simulink model "Navigation_Real"  (R2024a)
settings: Solver=VariableStepAuto  StartTime=0.0  StopTime=10.0  RelTol=1e-3
undefined symbols (not defined in the file or in its folder): Desired_Year_IGRF, Velocity_Ship_Mean
libraries: simulink_extras x4, sensorgpslib x1, sensorinslib x1
settings Model: Creator=gerar  LastModifiedBy=gerar

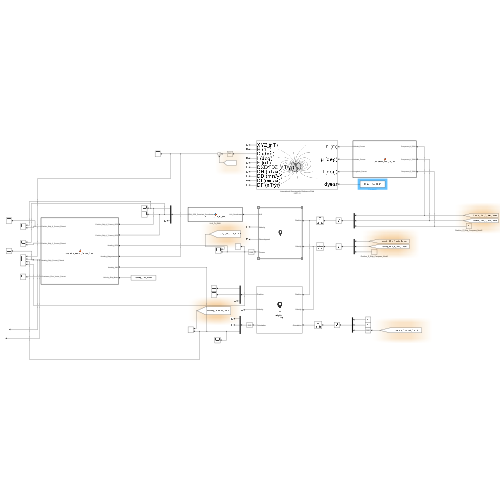
[thumbnail: Simulink's stored preview of the top-level diagram]
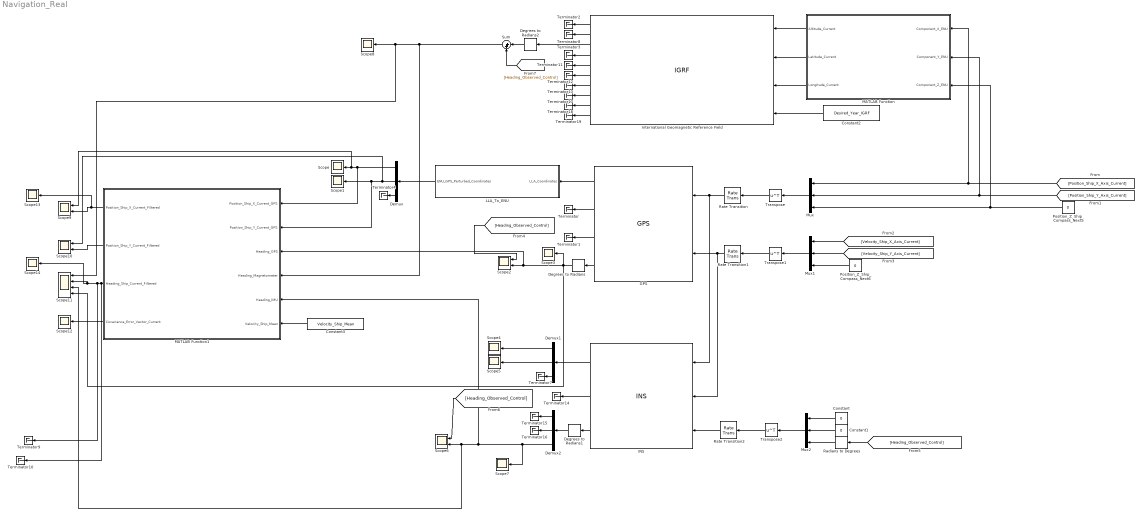
== system Navigation_Real ==
  Constant : Constant  Value=0
  Constant1 : Constant  Value=0
  Constant2 : Constant  Value=Desired_Year_IGRF
  Constant3 : Constant  Value=Velocity_Ship_Mean
  Degrees to Radians : simulink_extras/Transformations/Degrees to Radians
  Degrees to Radians1 : simulink_extras/Transformations/Degrees to Radians
  Degrees to Radians2 : simulink_extras/Transformations/Degrees to Radians
  Demux : Demux  Outputs=3
  Demux1 : Demux  Outputs=3
  Demux2 : Demux  Outputs=3
  GPS : sensorgpslib/GPS  DispRefFrame=ENU  PositionInputFormat=Local  ReferenceLocation=[43.059023, 3.002915 ,0]  HorizontalPositionAccuracy=1.6  VerticalPositionAccuracy=3  VelocityAccuracy=0.1  DecayFactor=0.999  SeedDouble=67  SimulateUsing=Interpreted execution
  INS : sensorinslib/INS  MountingLocation=[0 0 0]  RollAccuracy=0.2  PitchAccuracy=0.2  YawAccuracy=1  PositionAccuracy=1  VelocityAccuracy=0.05  UseAccelAndAngVel=off  AccelerationAccuracy=0  AngularVelocityAccuracy=0  TimeInput=off  PositionErrorFactor=[0 0 0]  SeedDouble=67  SimulateUsing=Code generation
  International Geomagnetic Reference Field : IGRF  month=January  day=1  year=2020
      settings: AttributesFormatString=%<generation>
  LLA_To_ENU : MATLAB Function  TreatAsAtomicUnit=on
  MATLAB Function : MATLAB Function  TreatAsAtomicUnit=on
  MATLAB Function1 : MATLAB Function  TreatAsAtomicUnit=on
  Mux : Mux  Inputs=3
  Mux1 : Mux  Inputs=3
  Mux2 : Mux  Inputs=3
  Position_Z_Ship_Compass_Next5 : Constant  Value=0
  Position_Z_Ship_Compass_Next6 : Constant  Value=0
  Radians to Degrees : simulink_extras/Transformations/Radians to Degrees
  Rate Transition : RateTransition  OutPortSampleTime=0.01
  Rate Transition1 : RateTransition  OutPortSampleTime=0.01
  Rate Transition2 : RateTransition  OutPortSampleTime=0.01
  Scope{,1,3..5,7..8,12..14} (10 alike) : Scope
  Scope{2,6,9..10} (4 alike) : Scope  NumInputPorts=2
  Scope11 : Scope  NumInputPorts=4
  Sum : Sum  Inputs=|++
  Terminator{,1..4,7..19} (18 alike) : Terminator
  Transpose : Math  Operator=transpose
  Transpose1 : Math  Operator=transpose
  Transpose2 : Math  Operator=transpose
  wires:
  MATLAB Function/1(Altitude_Current) -> International Geomagnetic Reference Field/1
  Demux/3 -> Terminator4/1
  International Geomagnetic Reference Field/6 -> Terminator12/1
  International Geomagnetic Reference Field/2 -> Terminator8/1
  Constant1/1 -> Mux2/2
  Transpose2/1 -> Rate Transition2/1
  Mux2/1 -> Transpose2/1
  Degrees to Radians1/1 -> Demux2/1
  [Heading_Observed_Control] -> Scope6/1
  MATLAB Function/3(Longitude_Current) -> International Geomagnetic Reference Field/3
  GPS/4 -> Degrees to Radians/1
  INS/3 -> Degrees to Radians1/1
  GPS/1 -> LLA_To_ENU/1(LLA_Coordinates)
  Demux1/1 -> Scope4/1
  Demux1/2 -> Scope5/1
  [Velocity_Ship_X_Axis_Current] -> Mux1/1
  Demux1/3 -> Terminator7/1
  [Position_Ship_Y_Axis_Current] -> MATLAB Function/2(Component_Y_ENU), Mux/2
  Degrees to Radians/1 -> MATLAB Function1/3(Heading_GPS), Scope2/2, Scope11/4, Scope3/1
  Demux/2 -> Scope10/1, MATLAB Function1/2(Position_Ship_Y_Current_GPS), Scope1/1
  [Heading_Observed_Control] -> Scope2/1
  Position_Z_Ship_Compass_Next6/1 -> Mux1/3
  Position_Z_Ship_Compass_Next5/1 -> MATLAB Function/3(Component_Z_ENU), Mux/3
  [Velocity_Ship_Y_Axis_Current] -> Mux1/2
  [Position_Ship_X_Axis_Current] -> MATLAB Function/1(Component_X_ENU), Mux/1
  Rate Transition/1 -> INS/1, GPS/1
  Transpose1/1 -> Rate Transition1/1
  International Geomagnetic Reference Field/3 -> Degrees to Radians2/1
  International Geomagnetic Reference Field/4 -> Terminator3/1
  International Geomagnetic Reference Field/9 -> Terminator18/1
  Rate Transition1/1 -> INS/2, GPS/2
  Constant/1 -> Mux2/1
  Mux/1 -> Transpose/1
  INS/2 -> Terminator14/1
  Sum/1 -> MATLAB Function1/4(Heading_Magnetometer), Scope11/1, Scope8/1
  [Heading_Observed_Control] -> Radians to Degrees/1
  International Geomagnetic Reference Field/7 -> Terminator13/1
  International Geomagnetic Reference Field/10 -> Terminator19/1
  International Geomagnetic Reference Field/8 -> Terminator17/1
  Demux2/2 -> Terminator16/1
  International Geomagnetic Reference Field/5 -> Terminator11/1
  International Geomagnetic Reference Field/1 -> Terminator2/1
  MATLAB Function/2(Latitude_Current) -> International Geomagnetic Reference Field/2
  Demux2/3 -> Scope7/1, Scope11/3, Scope6/2, MATLAB Function1/5(Heading_IMU)
  Transpose/1 -> Rate Transition/1
  INS/1 -> Demux1/1
  Demux/1 -> MATLAB Function1/1(Position_Ship_X_Current_GPS), Scope9/1, Scope/1
  Degrees to Radians2/1 -> Sum/1
  GPS/3 -> Terminator1/1
  Constant2/1 -> International Geomagnetic Reference Field/4
  Radians to Degrees/1 -> Mux2/3
  LLA_To_ENU/1(ENU_GPS_Perturbed_Coordinates) -> Demux/1
  MATLAB Function1/4(Covariance_Error_Vector_Current) -> Scope12/1
  Rate Transition2/1 -> INS/3
  Demux2/1 -> Terminator15/1
  GPS/2 -> Terminator/1
  MATLAB Function1/2(Position_Ship_Y_Current_Filtered) -> Scope10/2
  Mux1/1 -> Transpose1/1
  Constant3/1 -> MATLAB Function1/6(Velocity_Ship_Mean)
  MATLAB Function1/1(Position_Ship_X_Current_Filtered) -> Scope13/1, Scope9/2
  [Heading_Observed_Control] -> Sum/2
  MATLAB Function1/3(Heading_Ship_Current_Filtered) -> Terminator10/1, Terminator9/1, Scope14/1, Scope11/2

== matlab function Navigation_Real/LLA_To_ENU ==
  data: LLA_Coordinates input; ENU_GPS_Perturbed_Coordinates output
function ENU_GPS_Perturbed_Coordinates = Conversion_LLA_To_ENU(LLA_Coordinates)

% Reference point:
Reference_Point_Port_Mahon = [43.059023,3.002915,0];
Semi_Major_Axis = 6378137.0;
Flattening = 1/298.25;

% This function serves as a mean to convert LLA coordinates to ENU
% coordinates:
ENU_GPS_Perturbed_Coordinates = LLA_To_ENU(LLA_Coordinates(1),LLA_Coordinates(2),LLA_Coordinates(3),...
                                           Reference_Point_Port_Mahon(1),Reference_Point_Port_Mahon(2),...
                                           Reference_Point_Port_Mahon(3),Semi_Major_Axis,Flattening);


end

== matlab function Navigation_Real/MATLAB Function ==
  data: Altitude_Current output; Latitude_Current output; Longitude_Current output; Component_X_ENU input; Component_Y_ENU input; Component_Z_ENU input
function [Altitude_Current,Latitude_Current,Longitude_Current] = Conversion_ENU_To_LAA(Component_X_ENU,...
                                                                                       Component_Y_ENU,...
                                                                                       Component_Z_ENU)

% This function serves as a mean to convert ENU coordinates into LLA
% coordinates. Need to write an embedded function to be injected in the
% Mission Software.
% Reference point for the current mission;
Reference_Point_Port_Mahon = [43.059023,3.002915,0];
Position_Vector_ENU_Current = [Component_X_ENU,Component_Y_ENU,Component_Z_ENU];

% Conversion using Matlab function:
Position_Vector_LLA_Current = enu2lla(Position_Vector_ENU_Current,Reference_Point_Port_Mahon,'ellipsoid');

% Feed the outputs:
Latitude_Current = Position_Vector_LLA_Current(1);
Altitude_Current = Position_Vector_LLA_Current(3);
Longitude_Current = Position_Vector_LLA_Current(2);

end

== matlab function Navigation_Real/MATLAB Function1 ==
  data: Position_Ship_X_Current_GPS input; Position_Ship_Y_Current_GPS input; Heading_GPS input; Heading_Magnetometer input; Heading_IMU input; Position_Ship_X_Current_Filtered output; Position_Ship_Y_Current_Filtered output; Heading_Ship_Current_Filtered output; Covariance_Error_Vector_Current output; Velocity_Ship_Mean input
function [Position_Ship_X_Current_Filtered,...
          Position_Ship_Y_Current_Filtered,...
          Heading_Ship_Current_Filtered,...
          Covariance_Error_Vector_Current]  = Navigation_Kalman_Sensor_Fusion(Position_Ship_X_Current_GPS,...
                                                                              Position_Ship_Y_Current_GPS,...
                                                                              Heading_GPS,...
                                                                              Heading_Magnetometer,...
                                                                              Heading_IMU,...
                                                                              Velocity_Ship_Mean)

% This function serves as a filterting and data fusion to provide the ship
% with the right heading data.

% Openwork modifications:
% - Include the position given by the IMU if needed.
% - Complexification of the state model.

% ----------------------------------------------------------------
% 1) Definition of the process model:
% ----------------------------------------------------------------
% We define the following process model state vector:
% States_Initial_Model = [Position_X_Current;...
%                   Position_Y_Current;...
%                   Psi_Heading_Current;...
%                   Velocity_Current];

% Initialization of the current models:
Position_Ship_X_Current_Model = Position_Ship_X_Current_GPS;
Position_Ship_Y_Current_Model = Position_Ship_Y_Current_GPS;
Heading_Current_Model = Heading_GPS;
Velocity_Ship_Model = Velocity_Ship_Mean;

States_Initial_Model = [Position_Ship_X_Current_Model;...
                        Position_Ship_Y_Current_Model;...
                        Heading_Current_Model;...
                        Velocity_Ship_Model];

% We then define the process noise covariance matrix refered as the 'Q'
% matrix in estimation. This has a link with how one is confident about the
% used model:
Variance_Position_X = 0.5;
Variance_Position_Y = 0.5;
Variance_Heading = (2*pi/180);
Variance_Velocity = 10e-4;
Process_Model_Covariance_Matrix = [Variance_Position_X^2 0 0 0;
                                   0 Variance_Position_Y^2 0 0;
                                   0 0 Variance_Heading^2 0;
                                   0 0 0 Variance_Velocity^2];

% We define the covariance matrix of the states at the initial step refered as the 'P0|0':
% We just take Covariance_Matrix_States_Initial_Model =
% Process_Model_Covariance_Matrix:
Covariance_States_Initial_Model = Process_Model_Covariance_Matrix;

% Define the control input matrix refered as the 'B' matrix in the usual
% description of linear state-space system reprezentation:
Control_Inputs_Initial = 0; % Process model considered as without input influence.

% Chose the step time, it shall be aligned with HW specification:
Time_Step_HW = 1;

% NOTA:
% When calling the EKF function such that Estimates = EKF(), to get the
% proper evaluated functions used inside (Jacobians for example), then use
% the notation Estimates = EKF(Jacobian(Variable1,Variable2)).
% If it's not working, then delete the function as an input of the EKF,
% call it directly inside the EKF function. But pay attention to get the
% good inputs inside the EKF function.
% /!\ Same thing for the Function_Process_Model inside the EKF /!\.

% ----------------------------------------------------------------
% 2) Measurement & Innovation model:
% ----------------------------------------------------------------
% We define the following measurement model state vector:
% Measurement_Vector = [Position_X_Current;...
%                       Position_Y_Current;...
%                       Psi_Heading_GNSS_Current;...
%                       Psi_Heading_Mag_Current;...
%                       Psi_Heading_IMU_Current
%                       Velocity_Current];

% Definition of the measurement noise covariance matrix refered as 'R' matrix:
% Retake the Variance_Position_X, Variance_Position_Y, Variance_Velocity
% and Variance_Heading for Variance_Heading_GNSS used in the process model section:
% To be aligned with the specification from the sensors and the models used
% for the Navigation:
Variance_Position_X_GPS = 1.5;
Variance_Position_Y_GPS = 1;
Variance_Heading_GNSS = 6*(pi/180);
Variance_Heading_Magnetic = 10*(pi/180);
Variance_Heading_IMU = 15*(pi/180);
Measurement_Covariance_Matrix = [Variance_Position_X_GPS 0 0 0 0 0;
                                 0 Variance_Position_Y_GPS 0 0 0 0;
                                 0 0 Variance_Heading_GNSS 0 0 0;
                                 0 0 0 Variance_Heading_Magnetic 0 0;
                                 0 0 0 0 Variance_Heading_IMU 0;
                                 0 0 0 0 0 Variance_Velocity];

% Define the measurement model matrix: (ofter refered as 'H' or 'Gx'
% matrices):
Measurement_Model_Matrix = [1 0 0 0;
                            0 1 0 0;
                            0 0 1 0;
                            0 0 1 0;
                            0 0 1 0;
                            0 0 0 1];

% ----------------------------------------------------------------
% Extended Kalman Filter loop calculations:
% ----------------------------------------------------------------
% Store the results:
% States_Estimated_EKF = [];
% Covariance_Estimated_EKF = [];

% Initialization:
States_Previous = States_Initial_Model; % The 'X' state vector.
Covariance_State_Previous = Covariance_States_Initial_Model; % The 'P0|0' equal to 'Q' in this case.
Control_Inputs_Previous = Control_Inputs_Initial; % The usual 'B' matrix but unused here.
Process_Model_Covariance_Matrix_Previous = Process_Model_Covariance_Matrix; % The 'Q' process model matrix.
Measurement_Covariance_Matrix_Previous = Measurement_Covariance_Matrix; % The 'R' measurement matrix.
Measurment_Current = [Position_Ship_X_Current_GPS,Position_Ship_Y_Current_GPS,Heading_GPS,Heading_Magnetometer,...
                      Heading_IMU,Velocity_Ship_Mean];

% EKF loop calculation:
[State_Aposteriori_Current,Covariance_Aposteriori_Current] = EKF_Heading(States_Previous,Covariance_State_Previous,Control_Inputs_Previous,...
                                                                         Jacobian_State_Process_Model(States_Previous(4),States_Previous(3),Time_Step_HW),...
                                                                         Process_Model_Covariance_Matrix_Previous,Measurement_Model_Matrix,...
                                                                         Measurement_Covariance_Matrix_Previous,...
                                                                         Function_Process_Model(States_Previous(1),States_Previous(2),States_Previous(3),States_Previous(4),Time_Step_HW),...
                                                                         Measurment_Current');


% Inputs update:
% States_Initial_Model = State_Aposteriori_Current;
% Covariance_States_Initial_Model = Covariance_Aposteriori_Current;

% % Store the results:
% States_Estimated_EKF = [States_Estimated_EKF,State_Aposteriori_Current];
% Covariance_Estimated_EKF = [Covariance_Estimated_EKF,Covariance_Aposteriori_Current];

% Store the interesting components of the covariance matrix (diagonal
% terms):
Covariance_Position_X = Covariance_Aposteriori_Current(1,1);
Covariance_Position_Y = Covariance_Aposteriori_Current(2,2);
Covariance_Psi_Heading = Covariance_Aposteriori_Current(3,3);
Covariance_Velocity = Covariance_Aposteriori_Current(4,4);
Covariance_Error_Vector_Current = [Covariance_Position_X;...
                                   Covariance_Position_Y;...
                                   Covariance_Psi_Heading;...
                                   Covariance_Velocity];

% Filtered and fused data:
Position_Ship_X_Current_Filtered = State_Aposteriori_Current(1);
Position_Ship_Y_Current_Filtered = State_Aposteriori_Current(2);
Heading_Ship_Current_Filtered = State_Aposteriori_Current(3);
Velocity_Current_Filtered = State_Aposteriori_Current(4); % The velocity is supposed constant.

end
